simulink model "test_source_value"  (R2017a)
settings: Solver=VariableStepAuto  StartTime=0.0  StopTime=10.0  RelTol=1e-3
undefined symbols (not defined in the file or in its folder): sys, x0
settings Model: Creator=brunolnetto  LastModifiedBy=brunolnetto

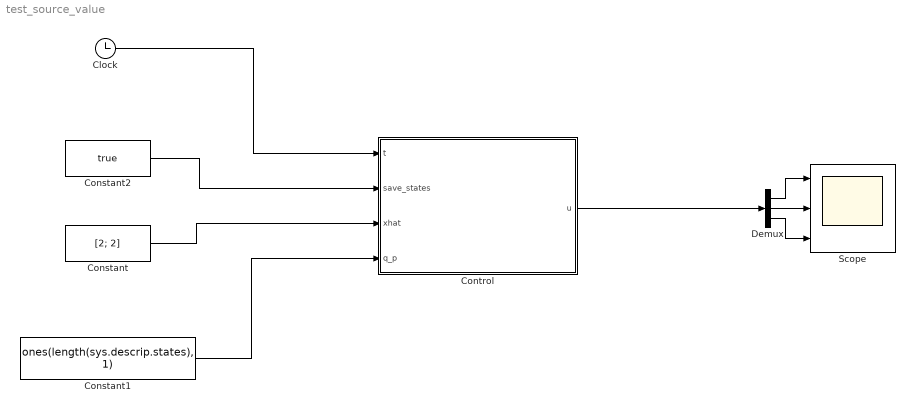
== system test_source_value ==
  Clock : Clock
  Constant : Constant  Value=[2; 2]
  Constant1 : Constant  Value=ones(length(sys.descrip.states), 1)
  Constant2 : Constant  Value=true
  Control : Subsystem
      mask Display: image('./controller.png');
  Demux : Demux  Outputs=3
  Scope : Scope  NumInputPorts=3
  wires:
  Constant/1 -> Control/3(xhat)
  Constant1/1 -> Control/4(q_p)
  Clock/1 -> Control/1(t)
  Constant2/1 -> Control/2(save_states)
  Control/1(u) -> Demux/1
  Demux/2 -> Scope/2
  Demux/1 -> Scope/1
  Demux/3 -> Scope/3

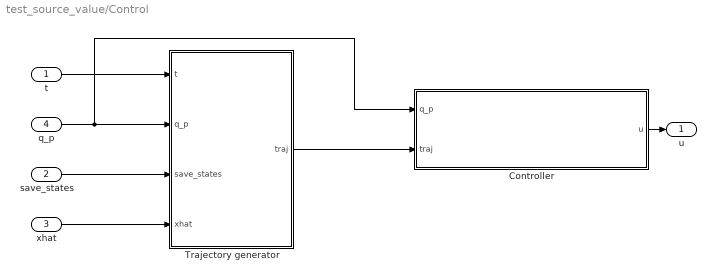
== system test_source_value/Control ==
  t : Inport
  save_states : Inport  Port=2
  xhat : Inport  Port=3
  q_p : Inport  Port=4
  Controller : Subsystem
      mask Display: image('./controller.png');
  Trajectory generator : Subsystem
  u : Outport
  wires:
  t/1 -> Trajectory generator/1(t)
  save_states/1 -> Trajectory generator/3(save_states)
  q_p/1 -> Controller/1(q_p), Trajectory generator/2(q_p)
  xhat/1 -> Trajectory generator/4(xhat)
  Controller/1(u) -> u/1
  Trajectory generator/1(traj) -> Controller/2(traj)

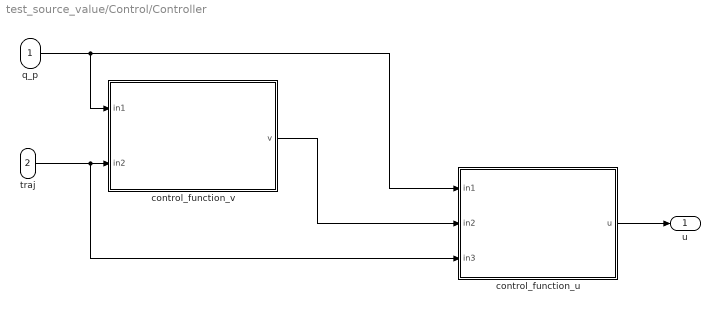
== system test_source_value/Control/Controller ==
  q_p : Inport
  traj : Inport  Port=2
  control_function_u : MATLAB Function  TreatAsAtomicUnit=on
  control_function_v : MATLAB Function  TreatAsAtomicUnit=on
  u : Outport
  wires:
  control_function_v/1(v) -> control_function_u/2(in2)
  q_p/1 -> control_function_v/1(in1), control_function_u/1(in1)
  control_function_u/1(u) -> u/1
  traj/1 -> control_function_u/3(in3), control_function_v/2(in2)

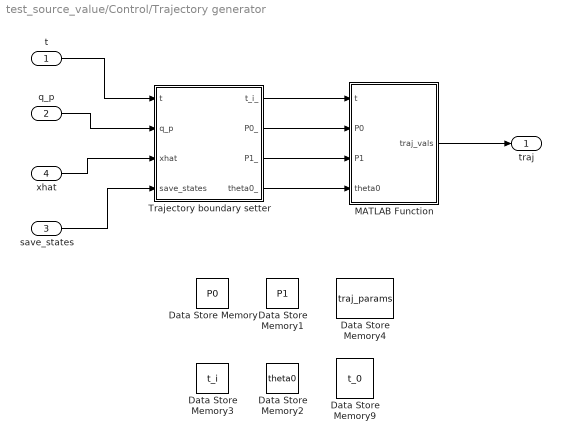
== system test_source_value/Control/Trajectory generator ==
  t : Inport
  q_p : Inport  Port=2
  save_states : Inport  Port=3
  xhat : Inport  Port=4
  Data Store Memory : DataStoreMemory  DataStoreName=P0  ReadBeforeWriteMsg=warning  WriteAfterWriteMsg=warning  WriteAfterReadMsg=warning  InitialValue=x0(1:2)  ShowAdditionalParam=off  OutDataTypeStr=double  Dimensions=[2, 1]
  Data Store Memory1 : DataStoreMemory  DataStoreName=P1  ReadBeforeWriteMsg=warning  WriteAfterWriteMsg=warning  WriteAfterReadMsg=warning  InitialValue=xhat0  ShowAdditionalParam=off  OutDataTypeStr=double
  Data Store Memory2 : DataStoreMemory  DataStoreName=theta0  ReadBeforeWriteMsg=warning  WriteAfterWriteMsg=warning  WriteAfterReadMsg=warning  InitialValue=x0(3)  ShowAdditionalParam=off  OutDataTypeStr=double
  Data Store Memory3 : DataStoreMemory  DataStoreName=t_i  ReadBeforeWriteMsg=warning  WriteAfterWriteMsg=warning  WriteAfterReadMsg=warning  ShowAdditionalParam=off  OutDataTypeStr=double
  Data Store Memory4 : DataStoreMemory  DataStoreName=traj_params  ReadBeforeWriteMsg=warning  WriteAfterWriteMsg=warning  WriteAfterReadMsg=warning  ShowAdditionalParam=off  OutDataTypeStr=double
  Data Store Memory9 : DataStoreMemory  DataStoreName=t_0  ReadBeforeWriteMsg=warning  WriteAfterWriteMsg=warning  WriteAfterReadMsg=warning  ShowAdditionalParam=off  OutDataTypeStr=double
  MATLAB Function : MATLAB Function  TreatAsAtomicUnit=on
  Trajectory boundary setter : MATLAB Function  TreatAsAtomicUnit=on
  traj : Outport
  wires:
  Trajectory boundary setter/4(theta0_) -> MATLAB Function/4(theta0)
  Trajectory boundary setter/2(P0_) -> MATLAB Function/2(P0)
  q_p/1 -> Trajectory boundary setter/2(q_p)
  MATLAB Function/1(traj_vals) -> traj/1
  t/1 -> Trajectory boundary setter/1(t)
  Trajectory boundary setter/3(P1_) -> MATLAB Function/3(P1)
  Trajectory boundary setter/1(t_i_) -> MATLAB Function/1(t)
  xhat/1 -> Trajectory boundary setter/3(xhat)
  save_states/1 -> Trajectory boundary setter/4(save_states)

== matlab function test_source_value/Control/Controller/control_function_u ==
  data: in1 input; u output; in2 input; in3 input
function u = ControlFunction_u(in1,in2,in3)

%    This function was generated by the Symbolic Math Toolbox version 7.2.

%    18-Feb-2021 10:17:31



p1 = in1(7,:);

p2 = in1(8,:);

p3 = in1(9,:);

th = in1(3,:);

th1 = in1(4,:);

th2 = in1(5,:);

th3 = in1(6,:);

v1 = in2(1,:);

v2 = in2(2,:);

v3 = in2(3,:);

x = in1(1,:);

y = in1(2,:);

y1_ref = in3(1,:);

y2_ref = in3(4,:);

y3_ref = in3(7,:);

yp1_ref = in3(2,:);

yp2_ref = in3(5,:);

yp3_ref = in3(8,:);

ypp1_ref = in3(3,:);

ypp2_ref = in3(6,:);

ypp3_ref = in3(9,:);

t2 = sin(th1);

t3 = sin(th2);

t4 = sin(th3);

t5 = t2.^2;

t6 = t5.*1.862411627770002e-9;

t7 = t3.^2;

t8 = t7.*1.862411627770002e-9;

t9 = t4.^2;

t10 = t9.*1.862411627770002e-9;

t11 = t6+t8+t10-1.044894955682166e-4;

t12 = 1.0./t11;

t13 = th+5.235987755982989e-1;

t14 = th+1.047197551196598;

t15 = sin(t14);

t16 = cos(t13);

t17 = cos(th);

t18 = sin(t13);

t19 = sin(th);

t20 = cos(t14);

t21 = p3.^2;

t22 = cos(th2);

t23 = cos(th3);

t24 = t12.*t15.*t18.*1.63236267389886e1;

t25 = t12.*t16.*t17.*1.63236267389886e1;

t26 = t12.*t19.*t20.*-1.63236267389886e1;

t27 = t12.*t15.*t17.*1.63236267389886e1;

t28 = t12.*t18.*t19.*1.63236267389886e1;

t29 = t12.*t16.*t20.*1.63236267389886e1;

t30 = t24+t25+t26+t27+t28+t29;

t31 = 1.0./t30;

t32 = cos(th1);

t33 = p3.*-2.0e1;

t34 = th.*-1.0e2;

t35 = y3_ref.*1.0e2;

t36 = yp3_ref.*2.0e1;

t37 = t32.^2;

t38 = t37.*1.164007267356251e62;

t39 = t22.^2;

t40 = t39.*1.164007267356251e62;

t41 = t23.^2;

t42 = t41.*1.164007267356251e62;

t43 = t38+t40+t42+6.530244270833333e66;

t44 = 1.0./t43;

t45 = th1.*2.0;

t46 = sin(t45);

t47 = t21.*t46.*1.691871028134086e62;

t48 = th2.*2.0;

t49 = sin(t48);

t50 = t21.*t49.*1.691871028134086e62;

t51 = th3.*2.0;

t52 = sin(t51);

t53 = t21.*t52.*1.691871028134086e62;

t54 = t21.*3.926713624160408e26;

t55 = p2.*p3.*t2.*t17.*t32.*2.706993645014537e63;

t56 = p1.*p3.*t3.*t17.*t22.*-2.344325264465624e63;

t57 = p2.*p3.*t3.*t17.*t22.*-1.353496822507269e63;

t58 = p1.*p3.*t4.*t17.*t23.*2.344325264465624e63;

t59 = p2.*p3.*t4.*t17.*t23.*-1.353496822507269e63;

t60 = p1.*p3.*t2.*t19.*t32.*-2.706993645014537e63;

t61 = p1.*p3.*t3.*t19.*t22.*1.353496822507269e63;

t62 = p2.*p3.*t3.*t19.*t22.*-2.344325264465624e63;

t63 = p1.*p3.*t4.*t19.*t23.*1.353496822507269e63;

t64 = p2.*p3.*t4.*t19.*t23.*2.344325264465624e63;

t65 = t47+t50+t53+t54+t55+t56+t57+t58+t59+t60+t61+t62+t63+t64;

t66 = t44.*t65.*1.0;

t67 = t33+t34+t35+t36+t66+v3+ypp3_ref;

t68 = p1.*-2.0e1;

t69 = x.*-1.0e2;

t70 = y1_ref.*1.0e2;

t71 = yp1_ref.*2.0e1;

t72 = t3.*t17.*t21.*t22.*6.008948770734595e-6;

t73 = t4.*t17.*t21.*t23.*-6.008948770734595e-6;

t74 = t2.*t19.*t21.*t32.*6.938536380660578e-6;

t75 = t3.*t19.*t21.*t22.*-3.469268190330289e-6;

t76 = t4.*t19.*t21.*t23.*-3.469268190330289e-6;

t77 = t68+t69+t70+t71+t72+t73+t74+t75+t76+v1+ypp1_ref;

t78 = t12.*t15.*5.924170616113744e-1;

t79 = p2.*-2.0e1;

t80 = y.*-1.0e2;

t81 = y2_ref.*1.0e2;

t82 = yp2_ref.*2.0e1;

t83 = t2.*t17.*t21.*t32.*-6.938536380660578e-6;

t84 = t3.*t17.*t21.*t22.*3.469268190330289e-6;

t85 = t4.*t17.*t21.*t23.*3.469268190330289e-6;

t86 = t3.*t19.*t21.*t22.*6.008948770734595e-6;

t87 = t4.*t19.*t21.*t23.*-6.008948770734595e-6;

t88 = t79+t80+t81+t82+t83+t84+t85+t86+t87+v2+ypp2_ref;

t89 = t12.*t16.*5.924170616113744e-1;

t90 = t12.*t18.*5.924170616113744e-1;

t91 = t12.*t17.*5.924170616113744e-1;

u = [t31.*t88.*(t78+t89).*-1.0+t31.*t77.*(t90-t12.*t20.*5.924170616113744e-1).*1.0+t31.*t67.*(t15.*t18.*7.592384529762141e2+t16.*t20.*7.592384529762141e2);t31.*t88.*(t78+t12.*t19.*5.924170616113744e-1)+t31.*t77.*(t91+t12.*t20.*5.924170616113744e-1)+t31.*t67.*(t15.*t17.*7.592384529762141e2-t19.*t20.*7.592384529762141e2);t31.*t77.*(t90+t91).*-1.0+t31.*t88.*(t89-t12.*t19.*5.924170616113744e-1)+t31.*t67.*(t16.*t17.*7.592384529762141e2+t18.*t19.*7.592384529762141e2)];

end

== matlab function test_source_value/Control/Trajectory generator/MATLAB Function ==
  data: t input; traj_vals output; P0 input; P1 input; theta0 input; trajectory_info parameter; t_0 data_store_memory
function traj_vals = traj_gen(t, P0, P1, theta0, trajectory_info)
    global t_0;

    % Origin and destiny
    P0 = double(P0);
    P1 = double(P1);    
    
    % Trajectory options
    T = trajectory_info.T_traj;
    trajectory_info.thetaA = theta0;
    deltas = trajectory_info.deltas;
    
    delta_x = deltas(1);
    delta_y = deltas(2);
    delta_th = deltas(3);
    
    alpha_ = (t - t_0)/T;
    x_y = P0 + alpha_*(P1 - P0);
    dx_y = (P1 - P0)/T;
    th = atan2(dx_y(2), dx_y(1));
    
    traj_vals = [x_y(1); dx_y(1); 0; ...
                 x_y(2); dx_y(2); 0; ...
                 th; 0; 0];
end

== matlab function test_source_value/Control/Trajectory generator/Trajectory boundary setter ==
  data: t_i_ output; P0_ output; P1_ output; theta0_ output; t input; q_p input; xhat input; save_states input; t_0 data_store_memory; P0 data_store_memory; P1 data_store_memory; theta0 data_store_memory
function [t_i_, P0_, P1_, theta0_] = trajectory(t, q_p, xhat, save_states)
    global P0 P1 t_0 theta0;
    
    % Initial and end trajectory points
    if(save_states)
        t_0 = t;
        
        P0 = q_p(1:2);
        P1 = xhat;
        
        theta0 = q_p(3);
        
        t_i = t - t_0;
    end
    
    % Save state points
    P0_ = P0;
    P1_ = P1;
    theta0_ = theta0;
    t_i_ = t - t_0;
end

== matlab function test_source_value/Control/Controller/control_function_v ==
  data: in1 input; v output; in2 input
function v = ControlFunction_v(in1,in2)

%    This function was generated by the Symbolic Math Toolbox version 7.2.

%    18-Feb-2021 10:17:31



p1 = in1(7,:);

p2 = in1(8,:);

p3 = in1(9,:);

th = in1(3,:);

x = in1(1,:);

y = in1(2,:);

y1_ref = in2(1,:);

y2_ref = in2(4,:);

y3_ref = in2(7,:);

yp1_ref = in2(2,:);

yp2_ref = in2(5,:);

yp3_ref = in2(8,:);

v = [p1.*-8.850851939315746-p2.*6.985979122817269e-15+p3.*1.151052501459392e-14+th.*2.300083815459809e-13-x.*8.58342113757929e1-y.*9.849696885097055e-14+y1_ref.*8.58342113757929e1+y2_ref.*9.849696885097055e-14-y3_ref.*2.300083815459809e-13+yp1_ref.*8.850851939315746+yp2_ref.*6.985979122817269e-15-yp3_ref.*1.151052501459392e-14;p1.*-6.868253630130176e-15+p2.*1.156663849679688+p3.*1.100049243381861e-29+th.*1.68269267210036e-28-x.*9.738779833488807e-14+y.*5.458045375779881e1+y1_ref.*9.738779833488807e-14-y2_ref.*5.458045375779881e1-y3_ref.*1.68269267210036e-28+yp1_ref.*6.868253630130176e-15-yp2_ref.*1.156663849679688-yp3_ref.*1.100049243381861e-29;p1.*-1.214546375378912e-14+p2.*3.053453109182706e-30-p3.*2.564117268763276+th.*3.880875224509013e1+x.*1.393151854064802e-13+y.*1.269366772871808e-28-y1_ref.*1.393151854064802e-13-y2_ref.*1.269366772871808e-28-y3_ref.*3.880875224509013e1+yp1_ref.*1.214546375378912e-14-yp2_ref.*3.053453109182706e-30+yp3_ref.*2.564117268763276];

end
